simulink model "AircraftB"  (Simulink 10.0)
settings: Solver=ode45  StartTime=0.0  StopTime=10.0  MaxStep=0.01  RelTol=1e-7  EnableMultiTasking=on
undefined symbols (not defined in the file): ac
libraries: simulink x1
settings Model: Creator=sg6510  LastModifiedBy=bhisma
settings DataIOCC: LimitDataPoints=on  SignalLoggingSaveFormat=ModelDataLogs
settings OptimizationCC: ExpressionDepthLimit=2147483647
settings DebuggingCC: SolverPrmCheckMsg=warning  FcnCallInpInsideContextMsg=warning  StateNameClashWarn=warning
settings ConfigComp: CovExternalEMLEnable=off

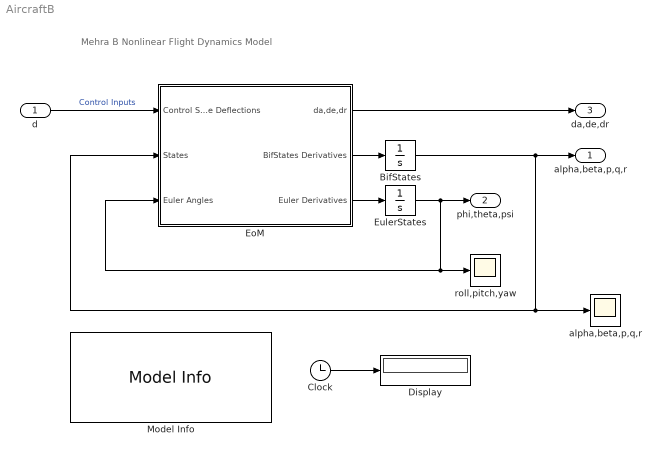
== system AircraftB ==
  note: Mehra B Nonlinear Flight Dynamics Model
  d : Inport
  BifStates : Integrator
  Clock : Clock
  Display : Display
  EoM : Subsystem  TreatAsAtomicUnit=on
      mask Display: image(imread('F100.jpg'),'center')
  EulerStates : Integrator
  Model Info : simulink/Model-Wide Utilities/Model Info  Frame=on  DisplayStringWithTags=|  HorizontalTextAlignment=Left  LeftAlignmentValue=0.02
      | Author: Steven Gill
      | Date: 28/01/2011
      | Modiefied:%<ModifiedDate>
      | Model Version:%<ModelVersion>
      | 
      | University of Bristol
  "alpha,beta,p,q,r " : Scope
  roll,pitch,yaw : Scope
  alpha,beta,p,q,r : Outport
  phi,theta,psi : Outport  Port=2
  da,de,dr : Outport  Port=3
  wires:
  EoM/2(BifStates Derivatives) -> BifStates/1
  BifStates/1 -> alpha,beta,p,q,r/1, EoM/2(States), "alpha,beta,p,q,r "/1
  d/1 -> EoM/1(Control Surface Deflections)  "Control Inputs"
  Clock/1 -> Display/1
  EoM/1(da,de,dr) -> da,de,dr/1
  EoM/3(Euler Derivatives) -> EulerStates/1
  EulerStates/1 -> phi,theta,psi/1, EoM/3(Euler Angles), roll,pitch,yaw/1

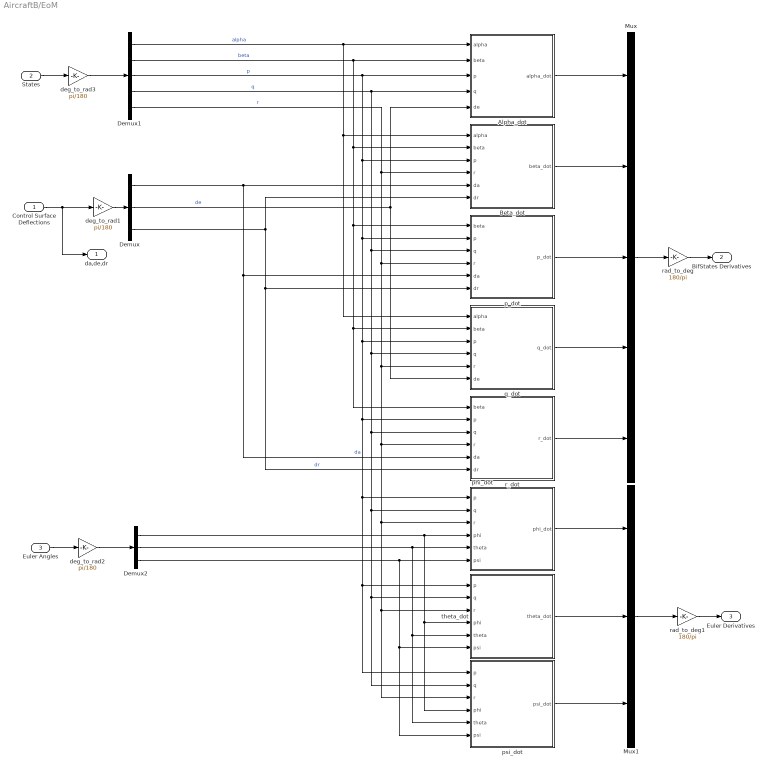
== system AircraftB/EoM ==
  Control Surface Deflections : Inport
  States : Inport  Port=2
  Euler Angles : Inport  Port=3
  Alpha_dot : Subsystem
  Beta_dot : Subsystem
  Demux : Demux  Outputs=3
  Demux1 : Demux  Outputs=5
  Demux2 : Demux  Outputs=3
  Mux : Mux  Inputs=5
  Mux1 : Mux  Inputs=3
  deg_to_rad1 : Gain  Gain=pi/180
  deg_to_rad2 : Gain  Gain=pi/180
  deg_to_rad3 : Gain  Gain=pi/180
  p_dot : Subsystem
  phi_dot : Subsystem
  psi_dot : Subsystem
  q_dot : Subsystem
  r_dot : Subsystem
  rad_to_deg : Gain  Gain=180/pi
  rad_to_deg1 : Gain  Gain=180/pi
  theta_dot : Subsystem
  da,de,dr : Outport
  BifStates Derivatives : Outport  Port=2
  Euler Derivatives : Outport  Port=3
  wires:
  Mux/1 -> rad_to_deg/1
  Control Surface Deflections/1 -> deg_to_rad1/1, da,de,dr/1
  States/1 -> deg_to_rad3/1
  Alpha_dot/1(alpha_dot) -> Mux/1
  Beta_dot/1(beta_dot) -> Mux/2
  p_dot/1(p_dot) -> Mux/3
  r_dot/1(r_dot) -> Mux/5
  q_dot/1(q_dot) -> Mux/4
  rad_to_deg/1 -> BifStates Derivatives/1
  deg_to_rad3/1 -> Demux1/1
  deg_to_rad1/1 -> Demux/1
  Demux1/1 -> Beta_dot/1(alpha), q_dot/1(alpha), Alpha_dot/1(alpha)  "alpha"
  Demux1/2 -> Alpha_dot/2(beta), r_dot/1(beta), q_dot/2(beta), p_dot/1(beta), Beta_dot/2(beta)  "beta"
  Demux1/3 -> Alpha_dot/3(p), Beta_dot/3(p), p_dot/2(p), q_dot/3(p), r_dot/2(p), psi_dot/1(p), theta_dot/1(p), phi_dot/1(p)  "p"
  Demux1/4 -> Alpha_dot/4(q), p_dot/3(q), q_dot/4(q), r_dot/3(q), psi_dot/2(q), theta_dot/2(q), phi_dot/2(q)  "q"
  Demux1/5 -> Beta_dot/4(r), p_dot/4(r), q_dot/5(r), r_dot/4(r), phi_dot/3(r), psi_dot/3(r), theta_dot/3(r)  "r"
  Demux/1 -> Beta_dot/5(da), r_dot/5(da), p_dot/5(da)  "da"
  Demux/2 -> q_dot/6(de), Alpha_dot/5(de)  "de"
  Demux/3 -> Beta_dot/6(dr), r_dot/6(dr), p_dot/6(dr)  "dr"
  phi_dot/1(phi_dot) -> Mux1/1
  theta_dot/1(theta_dot) -> Mux1/2
  psi_dot/1(psi_dot) -> Mux1/3
  Mux1/1 -> rad_to_deg1/1
  rad_to_deg1/1 -> Euler Derivatives/1
  Euler Angles/1 -> deg_to_rad2/1
  deg_to_rad2/1 -> Demux2/1
  Demux2/1 -> phi_dot/4(phi), psi_dot/4(phi), theta_dot/4(phi)
  Demux2/2 -> phi_dot/5(theta), psi_dot/5(theta), theta_dot/5(theta)
  Demux2/3 -> phi_dot/6(psi), psi_dot/6(psi), theta_dot/6(psi)

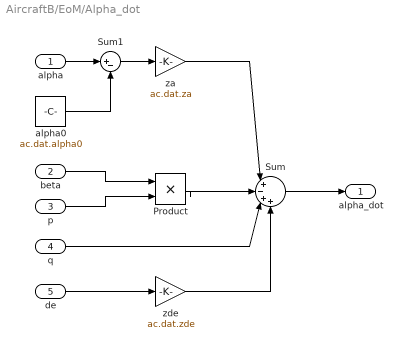
== system AircraftB/EoM/Alpha_dot ==
  alpha : Inport
  beta : Inport  Port=2
  p : Inport  Port=3
  q : Inport  Port=4
  de : Inport  Port=5
  Product : Product  RndMeth=Zero
  Sum : Sum  Inputs=|+-++
  Sum1 : Sum  Inputs=|+-
  alpha0 : Constant  Value=ac.dat.alpha0
  za : Gain  Gain=ac.dat.za
  zde : Gain  Gain=ac.dat.zde
  alpha_dot : Outport
  wires:
  Sum/1 -> alpha_dot/1
  Product/1 -> Sum/2
  beta/1 -> Product/1
  p/1 -> Product/2
  za/1 -> Sum/1
  q/1 -> Sum/3
  zde/1 -> Sum/4
  de/1 -> zde/1
  alpha/1 -> Sum1/1
  Sum1/1 -> za/1
  alpha0/1 -> Sum1/2

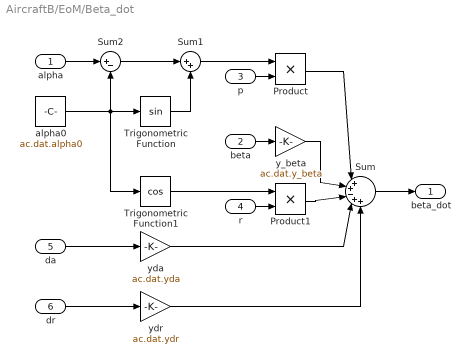
== system AircraftB/EoM/Beta_dot ==
  alpha : Inport
  beta : Inport  Port=2
  p : Inport  Port=3
  r : Inport  Port=4
  da : Inport  Port=5
  dr : Inport  Port=6
  Product : Product  RndMeth=Zero
  Product1 : Product  RndMeth=Zero
  Sum : Sum  Inputs=|++-++
  Sum1 : Sum  Inputs=|++
  Sum2 : Sum  Inputs=|+-
  Trigonometric Function : Trigonometry
  Trigonometric Function1 : Trigonometry  Operator=cos
  alpha0 : Constant  Value=ac.dat.alpha0
  y_beta : Gain  Gain=ac.dat.y_beta
  yda : Gain  Gain=ac.dat.yda
  ydr : Gain  Gain=ac.dat.ydr
  beta_dot : Outport
  wires:
  Sum/1 -> beta_dot/1
  beta/1 -> y_beta/1
  y_beta/1 -> Sum/2
  p/1 -> Product/2
  Product/1 -> Sum/1
  Sum1/1 -> Product/1
  da/1 -> yda/1
  dr/1 -> ydr/1
  alpha/1 -> Sum2/1
  alpha0/1 -> Sum2/2, Trigonometric Function/1, Trigonometric Function1/1
  Sum2/1 -> Sum1/1
  Trigonometric Function/1 -> Sum1/2
  r/1 -> Product1/2
  Trigonometric Function1/1 -> Product1/1
  Product1/1 -> Sum/3
  yda/1 -> Sum/4
  ydr/1 -> Sum/5

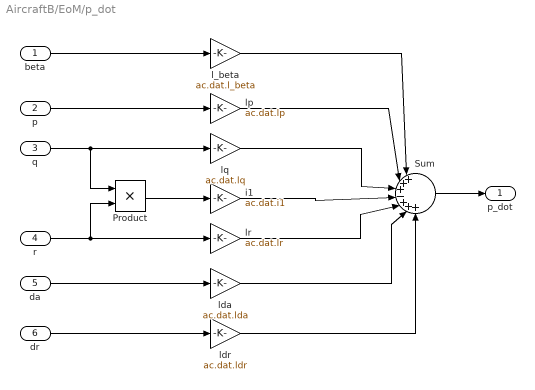
== system AircraftB/EoM/p_dot ==
  beta : Inport
  p : Inport  Port=2
  q : Inport  Port=3
  r : Inport  Port=4
  da : Inport  Port=5
  dr : Inport  Port=6
  Product : Product  RndMeth=Zero
  Sum : Sum  Inputs=|+++-+++
  i1 : Gain  Gain=ac.dat.i1
  l_beta : Gain  Gain=ac.dat.l_beta
  lda : Gain  Gain=ac.dat.lda
  ldr : Gain  Gain=ac.dat.ldr
  lp : Gain  Gain=ac.dat.lp
  lq : Gain  Gain=ac.dat.lq
  lr : Gain  Gain=ac.dat.lr
  p_dot : Outport
  wires:
  Sum/1 -> p_dot/1
  beta/1 -> l_beta/1
  q/1 -> lq/1, Product/1
  r/1 -> lr/1, Product/2
  p/1 -> lp/1
  Product/1 -> i1/1
  da/1 -> lda/1
  dr/1 -> ldr/1
  l_beta/1 -> Sum/1
  lp/1 -> Sum/2
  lq/1 -> Sum/3
  i1/1 -> Sum/4
  lr/1 -> Sum/5
  lda/1 -> Sum/6
  ldr/1 -> Sum/7

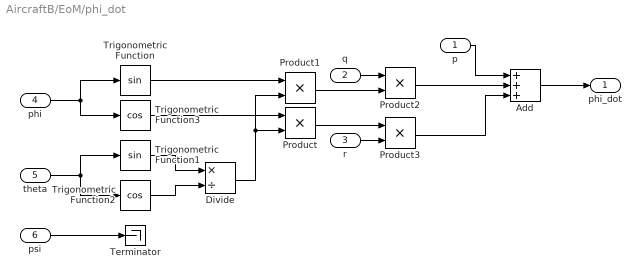
== system AircraftB/EoM/phi_dot ==
  p : Inport
  q : Inport  Port=2
  r : Inport  Port=3
  phi : Inport  Port=4
  theta : Inport  Port=5
  psi : Inport  Port=6
  Add : Sum  Inputs=+++
  Divide : Product  Inputs=*/
  Product{,1..3} (4 alike) : Product  RndMeth=Zero
  Terminator : Terminator
  Trigonometric Function : Trigonometry
  Trigonometric Function1 : Trigonometry
  Trigonometric Function2 : Trigonometry  Operator=cos
  Trigonometric Function3 : Trigonometry  Operator=cos
  phi_dot : Outport
  wires:
  Add/1 -> phi_dot/1
  phi/1 -> Trigonometric Function/1, Trigonometric Function3/1
  psi/1 -> Terminator/1
  theta/1 -> Trigonometric Function1/1, Trigonometric Function2/1
  Trigonometric Function1/1 -> Divide/1
  Trigonometric Function2/1 -> Divide/2
  Divide/1 -> Product/2, Product1/2
  Trigonometric Function3/1 -> Product/1
  Trigonometric Function/1 -> Product1/1
  q/1 -> Product2/1
  Product1/1 -> Product2/2
  Product/1 -> Product3/1
  r/1 -> Product3/2
  p/1 -> Add/1
  Product2/1 -> Add/2
  Product3/1 -> Add/3

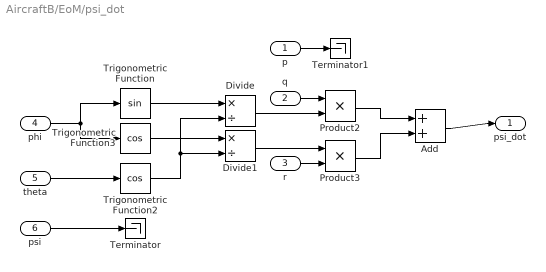
== system AircraftB/EoM/psi_dot ==
  p : Inport
  q : Inport  Port=2
  r : Inport  Port=3
  phi : Inport  Port=4
  theta : Inport  Port=5
  psi : Inport  Port=6
  Add : Sum
  Divide : Product  Inputs=*/
  Divide1 : Product  Inputs=*/
  Product2 : Product  RndMeth=Zero
  Product3 : Product  RndMeth=Zero
  Terminator : Terminator
  Terminator1 : Terminator
  Trigonometric Function : Trigonometry
  Trigonometric Function2 : Trigonometry  Operator=cos
  Trigonometric Function3 : Trigonometry  Operator=cos
  psi_dot : Outport
  wires:
  Add/1 -> psi_dot/1
  phi/1 -> Trigonometric Function/1, Trigonometric Function3/1
  psi/1 -> Terminator/1
  theta/1 -> Trigonometric Function2/1
  q/1 -> Product2/1
  r/1 -> Product3/2
  Trigonometric Function/1 -> Divide/1
  Trigonometric Function2/1 -> Divide/2, Divide1/2
  Trigonometric Function3/1 -> Divide1/1
  Divide/1 -> Product2/2
  Divide1/1 -> Product3/1
  p/1 -> Terminator1/1
  Product2/1 -> Add/1
  Product3/1 -> Add/2

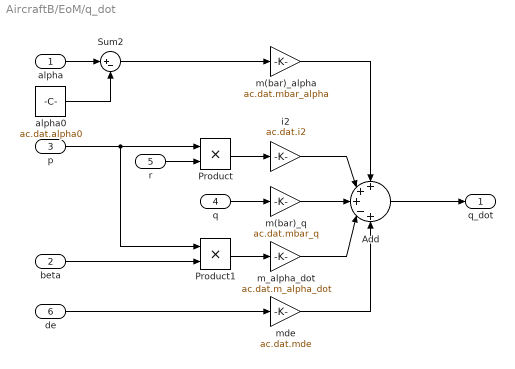
== system AircraftB/EoM/q_dot ==
  alpha : Inport
  beta : Inport  Port=2
  p : Inport  Port=3
  q : Inport  Port=4
  r : Inport  Port=5
  de : Inport  Port=6
  Add : Sum  Inputs=+++-+
  Product : Product  RndMeth=Zero
  Product1 : Product  RndMeth=Zero
  Sum2 : Sum  Inputs=|+-
  alpha0 : Constant  Value=ac.dat.alpha0
  i2 : Gain  Gain=ac.dat.i2
  m(bar)_alpha : Gain  Gain=ac.dat.mbar_alpha
  m(bar)_q : Gain  Gain=ac.dat.mbar_q
  m_alpha_dot : Gain  Gain=ac.dat.m_alpha_dot
  mde : Gain  Gain=ac.dat.mde
  q_dot : Outport
  wires:
  q/1 -> m(bar)_q/1
  Product/1 -> i2/1
  p/1 -> Product/1, Product1/1
  r/1 -> Product/2
  de/1 -> mde/1
  Product1/1 -> m_alpha_dot/1
  beta/1 -> Product1/2
  m(bar)_alpha/1 -> Add/1
  i2/1 -> Add/2
  m(bar)_q/1 -> Add/3
  m_alpha_dot/1 -> Add/4
  mde/1 -> Add/5
  Add/1 -> q_dot/1
  alpha/1 -> Sum2/1
  alpha0/1 -> Sum2/2
  Sum2/1 -> m(bar)_alpha/1

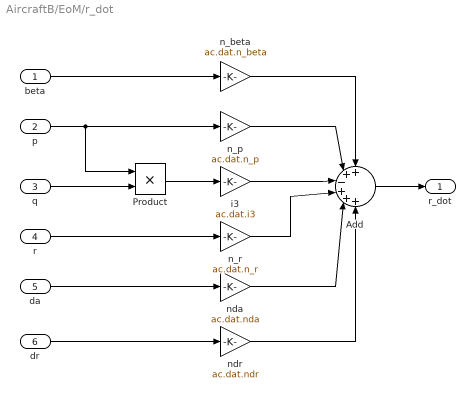
== system AircraftB/EoM/r_dot ==
  beta : Inport
  p : Inport  Port=2
  q : Inport  Port=3
  r : Inport  Port=4
  da : Inport  Port=5
  dr : Inport  Port=6
  Add : Sum  Inputs=++-+++
  Product : Product  RndMeth=Zero
  i3 : Gain  Gain=ac.dat.i3
  n_beta : Gain  Gain=ac.dat.n_beta
  n_p : Gain  Gain=ac.dat.n_p
  n_r : Gain  Gain=ac.dat.n_r
  nda : Gain  Gain=ac.dat.nda
  ndr : Gain  Gain=ac.dat.ndr
  r_dot : Outport
  wires:
  beta/1 -> n_beta/1
  p/1 -> n_p/1, Product/1
  r/1 -> n_r/1
  Product/1 -> i3/1
  q/1 -> Product/2
  da/1 -> nda/1
  dr/1 -> ndr/1
  n_beta/1 -> Add/1
  n_p/1 -> Add/2
  i3/1 -> Add/3
  n_r/1 -> Add/4
  nda/1 -> Add/5
  ndr/1 -> Add/6
  Add/1 -> r_dot/1

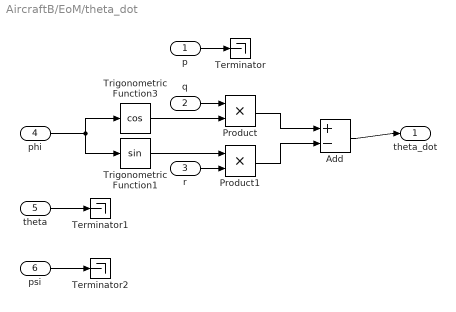
== system AircraftB/EoM/theta_dot ==
  p : Inport
  q : Inport  Port=2
  r : Inport  Port=3
  phi : Inport  Port=4
  theta : Inport  Port=5
  psi : Inport  Port=6
  Add : Sum  Inputs=+-
  Product : Product  RndMeth=Zero
  Product1 : Product  RndMeth=Zero
  Terminator : Terminator
  Terminator1 : Terminator
  Terminator2 : Terminator
  Trigonometric Function1 : Trigonometry
  Trigonometric Function3 : Trigonometry  Operator=cos
  theta_dot : Outport
  wires:
  Add/1 -> theta_dot/1
  r/1 -> Product1/2
  phi/1 -> Trigonometric Function3/1, Trigonometric Function1/1
  p/1 -> Terminator/1
  Trigonometric Function3/1 -> Product/2
  q/1 -> Product/1
  Trigonometric Function1/1 -> Product1/1
  theta/1 -> Terminator1/1
  psi/1 -> Terminator2/1
  Product/1 -> Add/1
  Product1/1 -> Add/2
